simulink model "assignment"  (R2024a)
settings: Solver=VariableStepAuto  StartTime=0.0  StopTime=10  RelTol=1e-3
undefined symbols (not defined in the file): A, B, C, h0, K, r
settings Model: Creator=HIEDA  LastModifiedBy=HIEDA

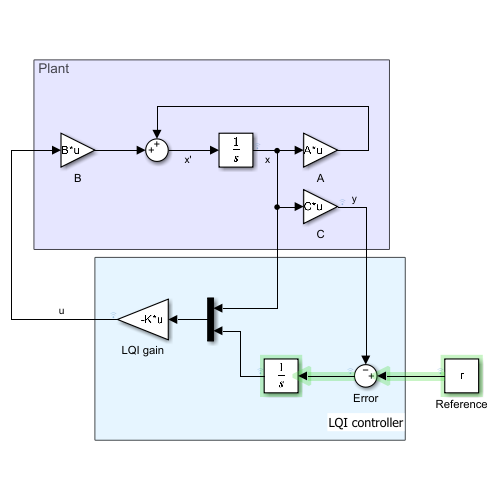
[thumbnail: Simulink's stored preview of the top-level diagram]
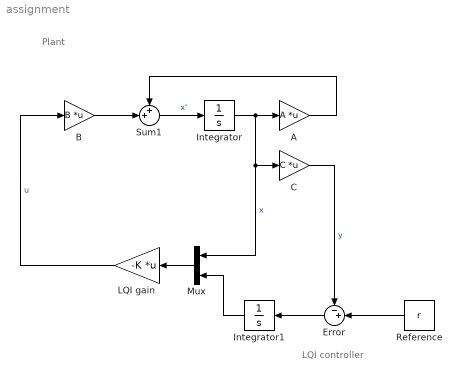
== system assignment ==
  note: LQI controller
  note: Plant
  A : Gain  Gain=A  Multiplication=Matrix(K*u)
  B : Gain  Gain=B  Multiplication=Matrix(K*u)
  C : Gain  Gain=C  Multiplication=Matrix(K*u)
  Error : Sum  Inputs=-+|
  Integrator : Integrator  InitialCondition=h0
  Integrator1 : Integrator
  LQI gain : Gain  Gain=-K  Multiplication=Matrix(K*u)
  Mux : Mux  Inputs=2
  Reference : Constant  Value=r  VectorParams1D=off
  Sum1 : Sum  Inputs=++|
  wires:
  C/1 -> Error/1  "y"
  B/1 -> Sum1/2
  A/1 -> Sum1/1
  Sum1/1 -> Integrator/1  "x'"
  Integrator/1 -> Mux/1, C/1, A/1  "x"
  Reference/1 -> Error/2
  Error/1 -> Integrator1/1
  LQI gain/1 -> B/1  "u"
  Integrator1/1 -> Mux/2
  Mux/1 -> LQI gain/1
